simulink model "Q3_sim"  (R2019b)
settings: Solver=VariableStepAuto  StartTime=0.0  StopTime=500  RelTol=1e-3
settings Model: Creator=Raj  LastModifiedBy=Raj

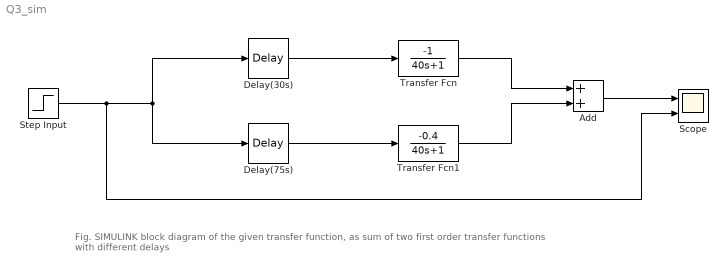
== system Q3_sim ==
  note: Fig. SIMULINK block diagram of the given transfer function, as sum of two first order transfer functions with different delays
  Add : Sum
  Delay(30s) : TransportDelay  DelayTime=30
  Delay(75s) : TransportDelay  DelayTime=75
  "Scope " : Scope  NumInputPorts=2
  "Step Input " : Step  Time=5  SampleTime=0
  Transfer Fcn : TransferFcn  Numerator=[-1]  Denominator=[40 1]
  Transfer Fcn1 : TransferFcn  Numerator=[-0.4]  Denominator=[40 1]
  wires:
  Delay(75s)/1 -> Transfer Fcn1/1
  Delay(30s)/1 -> Transfer Fcn/1
  "Step Input "/1 -> "Scope "/2, Delay(30s)/1, Delay(75s)/1
  Transfer Fcn/1 -> Add/1
  Transfer Fcn1/1 -> Add/2
  Add/1 -> "Scope "/1
